simulink library "mbed_targets_stm_nucleo_f303k8"  (R2015a)
settings: Solver=ode45  StartTime=0.0  StopTime=10.0  RelTol=1e-3
libraries: mbed_lib x3
settings Model: CovSFcnEnable=off  Creator=oh  LastModifiedBy=oh
settings DebuggingCC: SolverPrmCheckMsg=warning

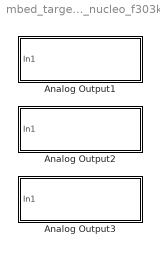
== system mbed_targets_stm_nucleo_f303k8 ==
  Analog Output1 : Subsystem  mask{Parameter1=0}
      mask Display:
      | offset=0.7;
      | plot([0+offset:0.025:0.25+offset],0.3*sin(2*pi*[0:0.1:1])+0.5)
      | port_label('input',1,['DAC1_1 (PA_4)']);
  Analog Output2 : Subsystem  mask{Parameter1=0}
      mask Display:
      | offset=0.7;
      | plot([0+offset:0.025:0.25+offset],0.3*sin(2*pi*[0:0.1:1])+0.5)
      | port_label('input',1,['DAC1_2 (PA_5)']);
  Analog Output3 : Subsystem  mask{Parameter1=0}
      mask Display:
      | offset=0.7;
      | plot([0+offset:0.025:0.25+offset],0.3*sin(2*pi*[0:0.1:1])+0.5)
      | port_label('input',1,['DAC2_1 (PA_6)']);

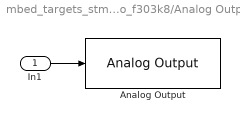
== system mbed_targets_stm_nucleo_f303k8/Analog Output1 ==
  In1 : Inport
  Analog Output : mbed_lib/GPIO/Analog Output  SParameter2=A  SParameter1=4  inputVariant=Double: 0 - 1.0f  SampleTime=-1
  wires:
  In1/1 -> Analog Output/1

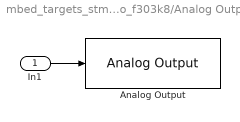
== system mbed_targets_stm_nucleo_f303k8/Analog Output2 ==
  In1 : Inport
  Analog Output : mbed_lib/GPIO/Analog Output  SParameter2=A  SParameter1=5  inputVariant=Double: 0 - 1.0f  SampleTime=-1
  wires:
  In1/1 -> Analog Output/1

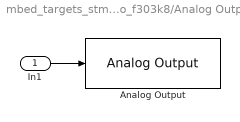
== system mbed_targets_stm_nucleo_f303k8/Analog Output3 ==
  In1 : Inport
  Analog Output : mbed_lib/GPIO/Analog Output  SParameter2=A  SParameter1=6  inputVariant=Double: 0 - 1.0f  SampleTime=-1
  wires:
  In1/1 -> Analog Output/1
